simulink model "untitled"  (R2016a)
settings: Solver=VariableStepAuto  StartTime=0.0  StopTime=1  RelTol=1e-3
libraries: SimscapeMacros x11, elec_lib x4, ProjectBlocks x3, fl_lib x1, nesl_utility x1, powerlib_meascontrol x1
settings Model: Creator=Peter  LastModifiedBy=Peter

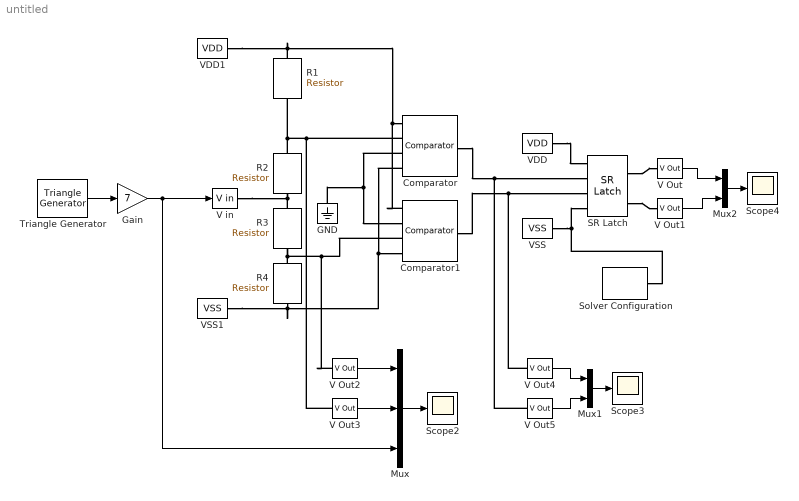
== system untitled ==
  Comparator : ProjectBlocks/Comparator
  Comparator1 : ProjectBlocks/Comparator
  GND : fl_lib/Electrical/Electrical Elements/Electrical Reference
  Gain : Gain  Gain=7
  Mux : Mux  Inputs=3
  Mux1 : Mux  Inputs=2
  Mux2 : Mux  Inputs=2
  R1 : elec_lib/Passive Devices/Resistor  R=10e3 Ohm  R_tol=5  enable_R_tol=0  tol_distribution=1  nSigma=4  enable_operating_limits=0  operating_limit_action=2  max_working_voltage=100 V  power_rating=1 W  enable_faults=0  fault_action=1  R_faulted=Inf Ohm  enable_temporal_fault=0  t_fault=1 s  enable_behavioral_fault=0  max_permissible_current=1 A  t_fail_on_current=1 s  noise_mode=0  sample_time=0.001 s  repeatability=1  auto_seed=1024917047  user_seed=0  Tdevice=25 degC  alpha=0.00393 1/K  Tmeas=25 degC  thermal_mass=100 J/K  initial_temperature=25 degC  power_derating_T1=70 degC  power_derating_T2=155 degC  operating_temperature_range_vec=[ -50 150 ] degC
  R2 : elec_lib/Passive Devices/Resistor  R=5e3 Ohm  R_tol=5  enable_R_tol=0  tol_distribution=1  nSigma=4  enable_operating_limits=0  operating_limit_action=2  max_working_voltage=100 V  power_rating=1 W  enable_faults=0  fault_action=1  R_faulted=Inf Ohm  enable_temporal_fault=0  t_fault=1 s  enable_behavioral_fault=0  max_permissible_current=1 A  t_fail_on_current=1 s  noise_mode=0  sample_time=0.001 s  repeatability=1  auto_seed=879328466  user_seed=0  Tdevice=25 degC  alpha=0.00393 1/K  Tmeas=25 degC  thermal_mass=100 J/K  initial_temperature=25 degC  power_derating_T1=70 degC  power_derating_T2=155 degC  operating_temperature_range_vec=[ -50 150 ] degC
  R3 : elec_lib/Passive Devices/Resistor  R=5e3 Ohm  R_tol=5  enable_R_tol=0  tol_distribution=1  nSigma=4  enable_operating_limits=0  operating_limit_action=2  max_working_voltage=100 V  power_rating=1 W  enable_faults=0  fault_action=1  R_faulted=Inf Ohm  enable_temporal_fault=0  t_fault=1 s  enable_behavioral_fault=0  max_permissible_current=1 A  t_fail_on_current=1 s  noise_mode=0  sample_time=0.001 s  repeatability=1  auto_seed=1110859295  user_seed=0  Tdevice=25 degC  alpha=0.00393 1/K  Tmeas=25 degC  thermal_mass=100 J/K  initial_temperature=25 degC  power_derating_T1=70 degC  power_derating_T2=155 degC  operating_temperature_range_vec=[ -50 150 ] degC
  R4 : elec_lib/Passive Devices/Resistor  R=10e3 Ohm  R_tol=5  enable_R_tol=0  tol_distribution=1  nSigma=4  enable_operating_limits=0  operating_limit_action=2  max_working_voltage=100 V  power_rating=1 W  enable_faults=0  fault_action=1  R_faulted=Inf Ohm  enable_temporal_fault=0  t_fault=1 s  enable_behavioral_fault=0  max_permissible_current=1 A  t_fail_on_current=1 s  noise_mode=0  sample_time=0.001 s  repeatability=1  auto_seed=3639188034  user_seed=0  Tdevice=25 degC  alpha=0.00393 1/K  Tmeas=25 degC  thermal_mass=100 J/K  initial_temperature=25 degC  power_derating_T1=70 degC  power_derating_T2=155 degC  operating_temperature_range_vec=[ -50 150 ] degC
  SR Latch : ProjectBlocks/SR Latch
  Scope2 : Scope
  Scope3 : Scope
  Scope4 : Scope
  Solver Configuration : nesl_utility/Solver Configuration  PhysicalDomain=network_engine_domain  SubClassName=solver  LeftPortType=input  RightPortType=generic  Accelerate=off  Tones=[]  Harmonics=[]  SimulateNoise=off  Profile=off  UseLocalSampling=off  EnableSwitchedLinearOptims=on  FrequencyDomain=off  UseCCode=off  RelTol=0.001  AbsTol=1e-06  MinStep=1e-09  ToWorkspace=off  RevertToSquareIcSolve=off  NumHomotopyIterations=100  PhasorMode=off  PhasorModeNumHarmonics=1  OverrideAbsTol=off  DoDC=off  ResidualTolerance=1e-09  UseLocalSolver=off  LocalSolverChoice=NE_BACKWARD_EULER_ADVANCER  LocalSolverSampleTime=0.001  DoFixedCost=off  MaxNonlinIter=3  MaxModeIter=2  LinearAlgebra=Sparse  DelaysMemoryBudget=1024  AutomaticFiltering=on  FilteringTimeConstant=0.001
  Triangle Generator : powerlib_meascontrol/Pulse & Signal Generators/Triangle Generator  Freq=3  Phase=90  Ts=0
  V Out{,1..5} (6 alike) : SimscapeMacros/V Out
  V in : SimscapeMacros/V in
  VDD : SimscapeMacros/VDD
  VDD1 : SimscapeMacros/VDD
  VSS : SimscapeMacros/VSS
  VSS1 : SimscapeMacros/VSS
  wires:
  V Out2/1 -> Mux/1
  V Out3/1 -> Mux/2
  Mux/1 -> Scope2/1
  V Out5/1 -> Mux1/2
  V Out4/1 -> Mux1/1
  Mux1/1 -> Scope3/1
  Mux2/1 -> Scope4/1
  V Out/1 -> Mux2/1
  V Out1/1 -> Mux2/2
  Triangle Generator/1 -> Gain/1
  Gain/1 -> Mux/3, V in/1
  connections:
  VSS/RConn1 -- SR Latch/LConn4 -- Solver Configuration/RConn1
  VDD/RConn1 -- SR Latch/LConn1
  SR Latch/RConn2 -- V Out1/LConn1
  SR Latch/RConn1 -- V Out/LConn1
  Comparator/RConn1 -- V Out5/LConn1 -- SR Latch/LConn2
  Comparator1/RConn1 -- SR Latch/LConn3 -- V Out4/LConn1
  VSS1/RConn1 -- R4/RConn1 -- Comparator/LConn4 -- Comparator1/LConn4
  VDD1/RConn1 -- R1/LConn1 -- Comparator1/LConn1 -- Comparator/LConn1
  Comparator/LConn3 -- GND/LConn1 -- Comparator1/LConn2
  R2/LConn1 -- V Out3/LConn1 -- Comparator/LConn2 -- R1/RConn1
  R3/LConn1 -- R2/RConn1 -- V in/RConn1
  R4/LConn1 -- V Out2/LConn1 -- Comparator1/LConn3 -- R3/RConn1
